simulink model "parte2"  (R2015a)
settings: Solver=ode3  StartTime=0.0  StopTime=39  RelTol=1e-3
values from neighbouring files (symbols this model uses):
  A = [2.83417400276 1 0 0 0 -3.24034029814 0 1 0 0 1.87807803148 0 ... (25 elements, 5x5)]    [16-10-2024-16-27-10_parte2_stepWithNoise.mat]    (also in 16-10-2024-17-42-48_parte2_Re10.mat; 16-10-2024-18-00-20_parte2_R1.mat; 16-10-2024-18-00-52_parte2_R1_G0_05.mat; 16-10-2024-18-02-38_parte2_R10_G0_05.mat)
  B = [1 0 0 0 0]    [16-10-2024-16-27-10_parte2_stepWithNoise.mat]    (also in 16-10-2024-17-42-48_parte2_Re10.mat; 16-10-2024-18-00-20_parte2_R1.mat; 16-10-2024-18-00-52_parte2_R1_G0_05.mat; 16-10-2024-18-02-38_parte2_R10_G0_05.mat)
  C = [17.301157538 -12.1905788706 0 0 0]    [16-10-2024-16-27-10_parte2_stepWithNoise.mat]    (also in 16-10-2024-17-42-48_parte2_Re10.mat; 16-10-2024-18-00-20_parte2_R1.mat; 16-10-2024-18-00-52_parte2_R1_G0_05.mat; 16-10-2024-18-02-38_parte2_R10_G0_05.mat)
  K = [1.48523121625 -2.43859165576 1.55399449774 -0.389429936703 -0.0278440976228]    [16-10-2024-16-27-10_parte2_stepWithNoise.mat]    (also in 16-10-2024-17-42-48_parte2_Re10.mat; 16-10-2024-18-00-20_parte2_R1.mat = [2.10722861971 -3.21463930579 1.86914882844 -0.438744538993 ; 16-10-2024-18-00-52_parte2_R1_G0_05.mat = [2.10722861971 -3.21463930579 1.86914882844 -0.438744538993 ; 16-10-2024-18-02-38_parte2_R10_G0_05.mat = [1.9592414811 -3.04091031101 1.80630248386 -0.429914029166 -)
  Ke = -2.55028399124    [16-10-2024-16-27-10_parte2_stepWithNoise.mat]    (also in 16-10-2024-17-42-48_parte2_Re10.mat; 16-10-2024-18-00-20_parte2_R1.mat; 16-10-2024-18-00-52_parte2_R1_G0_05.mat; 16-10-2024-18-02-38_parte2_R10_G0_05.mat)
  Kp = 35.0251781473    [16-10-2024-16-27-10_parte2_stepWithNoise.mat]    (also in 16-10-2024-17-42-48_parte2_Re10.mat; 16-10-2024-18-00-20_parte2_R1.mat; 16-10-2024-18-00-52_parte2_R1_G0_05.mat; 16-10-2024-18-02-38_parte2_R10_G0_05.mat)
  M = [0.0575697353703 0.00185632744036 -0.00164161433974 0.000565795375829 0.000246890631738]    [16-10-2024-16-27-10_parte2_stepWithNoise.mat]    (also in 16-10-2024-17-42-48_parte2_Re10.mat = [0.0563267449362 0.00846922395123 -0.00366362957776 -0.00060; 16-10-2024-18-00-20_parte2_R1.mat; 16-10-2024-18-00-52_parte2_R1_G0_05.mat; 16-10-2024-18-02-38_parte2_R10_G0_05.mat)
  Nbar = 0.0358785248867    [16-10-2024-16-27-10_parte2_stepWithNoise.mat]    (also in 16-10-2024-17-42-48_parte2_Re10.mat; 16-10-2024-18-00-20_parte2_R1.mat = 0.0569679861987; 16-10-2024-18-00-52_parte2_R1_G0_05.mat = 0.0569679861987; 16-10-2024-18-02-38_parte2_R10_G0_05.mat = 0.0515816294891)
  sampling_time = 0.02    [16-10-2024-16-27-10_parte2_stepWithNoise.mat]    (also in 16-10-2024-17-42-48_parte2_Re10.mat; 16-10-2024-18-00-20_parte2_R1.mat; 16-10-2024-18-00-52_parte2_R1_G0_05.mat; 16-10-2024-18-02-38_parte2_R10_G0_05.mat)
undefined symbols (not defined in the file or in its folder): MIO, National_Instruments, PCI
libraries: sldrtlib x3
settings Model: SimulationMode=external  ExtModeTrigDuration=300000  Creator=Alunos  LastModifiedBy=Alunos
settings HardwareCC: ProdIntDivRoundTo=Zero  ProdEndianess=LittleEndian  ProdHWDeviceType=Intel->x86/Pentium  TargetIntDivRoundTo=Zero  TargetEndianess=LittleEndian  TargetHWDeviceType=Intel->x86/Pentium
settings RTWCC: SystemTargetFile=rtwin.tlc  TemplateMakefile=rtwin.tmf  Description=Simulink Desktop Real-Time  RTWCompilerOptimization=on
settings CodeAppCC: MaxIdLength=95
settings RTWinTargetCC: TargetPreCompLibLocation=C:\Program Files\MATLAB\R2015a\toolbox\sldrt\lib\win32

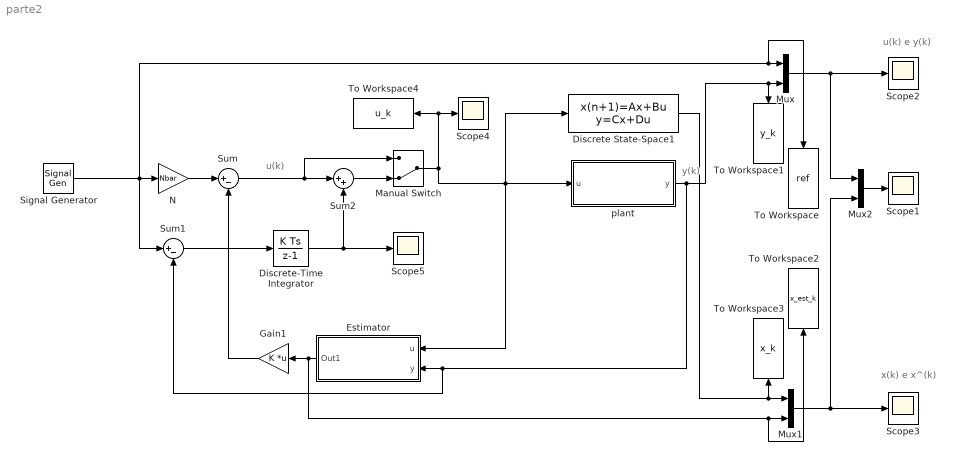
== system parte2 ==
  note: y(k)
  note: x(k) e x^(k)
  note: u(k) e y(k)
  note: u(k)
  Discrete State-Space1 : DiscreteStateSpace  A=A  B=B  C=ones(size(C))  D=0  SampleTime=sampling_time
  Discrete-Time Integrator : DiscreteIntegrator  gainval=0.1  InitialConditionSetting=State (most efficient)  SampleTime=sampling_time  UpperSaturationLimit=5  LowerSaturationLimit=-5
  Estimator : Subsystem
  Gain1 : Gain  Gain=K  Multiplication=Matrix(K*u)
  Manual Switch : ManualSwitch  CurrentSetting=0
  Mux : Mux  Inputs=2
  Mux1 : Mux  Inputs=2
  Mux2 : Mux  Inputs=2
  N : Gain  Gain=Nbar
  Scope{1..5} (5 alike) : Scope
      Scope1 settings: YMin=-525  YMax=0
      Scope2 settings: YMin=-50  YMax=45
      Scope3 settings: YMin=-525  YMax=0  SaveName=ScopeData2
      Scope4 settings: YMin=-0.5  YMax=2.5  SaveName=ScopeData3
      Scope5 settings: YMin=-10.75  YMax=-7.25  SaveName=ScopeData4
  Signal Generator : SignalGenerator  WaveForm=square  Amplitude=45  Frequency=0.05
  Sum : Sum  Inputs=|+-
  Sum1 : Sum  Inputs=|+-
  Sum2 : Sum  Inputs=|++
  To Workspace : ToWorkspace  VariableName=ref  SaveFormat=Structure With Time  SampleTime=sampling_time
  To Workspace1 : ToWorkspace  VariableName=y_k  SaveFormat=Structure With Time  SampleTime=sampling_time
  "To Workspace2 " : ToWorkspace  VariableName=x_est_k  SaveFormat=Structure With Time  SampleTime=sampling_time
  To Workspace3 : ToWorkspace  VariableName=x_k  SaveFormat=Structure With Time  SampleTime=sampling_time
  To Workspace4 : ToWorkspace  VariableName=u_k  SaveFormat=Structure With Time  SampleTime=sampling_time
  plant : Subsystem
  wires:
  Signal Generator/1 -> Sum1/1, To Workspace/1, Mux/1, N/1
  Estimator/1(Out1) -> Mux1/2, "To Workspace2 "/1, Gain1/1
  N/1 -> Sum/1
  Gain1/1 -> Sum/2
  Sum/1 -> Manual Switch/1, Sum2/1
  Discrete State-Space1/1 -> Mux1/1, To Workspace3/1
  Mux/1 -> Mux2/1, Scope2/1
  Mux1/1 -> Mux2/2, Scope3/1
  Mux2/1 -> Scope1/1
  plant/1("y ") -> Sum1/2, Estimator/2(y), Mux/2, To Workspace1/1
  Manual Switch/1 -> Estimator/1("u "), plant/1("u "), Discrete State-Space1/1, To Workspace4/1, Scope4/1
  Discrete-Time Integrator/1 -> Scope5/1, Sum2/2
  Sum2/1 -> Manual Switch/2
  Sum1/1 -> Discrete-Time Integrator/1

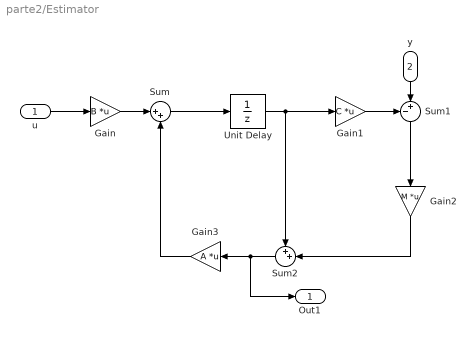
== system parte2/Estimator ==
  "u " : Inport
  y : Inport  Port=2
  Gain : Gain  Gain=B  Multiplication=Matrix(K*u)
  Gain1 : Gain  Gain=C  Multiplication=Matrix(K*u)
  Gain2 : Gain  Gain=M  Multiplication=Matrix(K*u)
  Gain3 : Gain  Gain=A  Multiplication=Matrix(K*u)
  Sum : Sum  Inputs=|++
  Sum1 : Sum  Inputs=-+|
  Sum2 : Sum  Inputs=++|
  Unit Delay : UnitDelay  SampleTime=sampling_time
  Out1 : Outport
  wires:
  y/1 -> Sum1/2
  Gain1/1 -> Sum1/1
  Sum1/1 -> Gain2/1
  Gain3/1 -> Sum/2
  Gain2/1 -> Sum2/2
  Sum2/1 -> Out1/1, Gain3/1
  Unit Delay/1 -> Sum2/1, Gain1/1
  Sum/1 -> Unit Delay/1
  Gain/1 -> Sum/1
  "u "/1 -> Gain/1

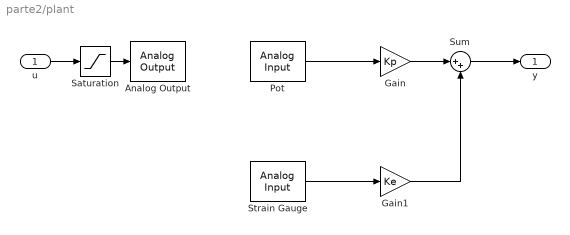
== system parte2/plant ==
  "u " : Inport
  Analog Output : sldrtlib/Analog Output  SampleTime=sampling_time  MaxMissedTicks=10  ShowMissedTicks=off  YieldWhenWaiting=off  DrvName=National_Instruments/PCI-MIO-16E-4  DrvAddress=4294967295  DrvOptions=[0 0 0 0 0 0]  Channels=1  RangeMode=1  VoltRange=1  InitialValue=0  FinalValue=0
      settings: AttributesFormatString=National Instruments\nPCI-MIO-16E-4 [auto]
  Gain : Gain  Gain=Kp
  Gain1 : Gain  Gain=Ke
  Pot : sldrtlib/Analog Input  SampleTime=sampling_time  MaxMissedTicks=10  ShowMissedTicks=off  YieldWhenWaiting=off  DrvName=National_Instruments/PCI-MIO-16E-4  DrvAddress=4294967295  DrvOptions=[0 0 0 0 0 0]  Channels=1  RangeMode=1  VoltRange=1  DataType=1
      settings: AttributesFormatString=National Instruments\nPCI-MIO-16E-4 [auto]
  Saturation : Saturate  UpperLimit=5  LowerLimit=-5
  Strain Gauge : sldrtlib/Analog Input  SampleTime=sampling_time  MaxMissedTicks=10  ShowMissedTicks=off  YieldWhenWaiting=off  DrvName=National_Instruments/PCI-MIO-16E-4  DrvAddress=4294967295  DrvOptions=[0 0 0 0 0 0]  Channels=2  RangeMode=1  VoltRange=1  DataType=1
      settings: AttributesFormatString=National Instruments\nPCI-MIO-16E-4 [auto]
  Sum : Sum  Inputs=|++
  "y " : Outport
  wires:
  Gain1/1 -> Sum/2
  Pot/1 -> Gain/1
  Strain Gauge/1 -> Gain1/1
  Gain/1 -> Sum/1
  Sum/1 -> "y "/1
  "u "/1 -> Saturation/1
  Saturation/1 -> Analog Output/1
